simulink model "simpleVehicleModel_Trial1"  (R2017b)
settings: Solver=FixedStepAuto  StartTime=0.0  StopTime=15  FixedStep=0.01  RelTol=1e-3
values from neighbouring files (symbols this model uses):
  beta_ref = 20*pi/180    (= 0.349065850399)    [initialize_simplemodel_Trial.m]
  g = 9.81    [initialize_simplemodel.m]    (also in initialize_simplemodel_Trial.m; tire_friction_circle.m)
  h = 0.35    [initialize_simplemodel.m]    (also in initialize_simplemodel_Trial.m)
  Izz = 1800    [initialize_simplemodel.m]    (also in initialize_simplemodel_Trial.m = 1400)
  lf = 1.4    [initialize_simplemodel.m]    (also in initialize_simplemodel_Trial.m)
  lr = 1.345    [initialize_simplemodel.m]    (also in initialize_simplemodel_Trial.m)
  m = 1400    [initialize_simplemodel.m]    (also in initialize_simplemodel_Trial.m = 1300; tire_friction_circle.m = 1300)
  r = 0.34    [initialize_simplemodel.m]    (also in initialize_simplemodel_Trial.m)
  tr = 1.684/2    (= 0.842)    [initialize_simplemodel.m]    (also in initialize_simplemodel_Trial.m)
  vx = 10    [initialize_simplemodel_Trial.m]    (also in pp_from_simple_model.m; tire_friction_circle.m = 5)
undefined symbols (not defined in the file or in its folder): DiscIntNeverNeededParam, G1, G2
libraries: simulink x49
(part 1 of 2)
settings Model: Creator=ashwin.ramanujam  LastModifiedBy=gandh

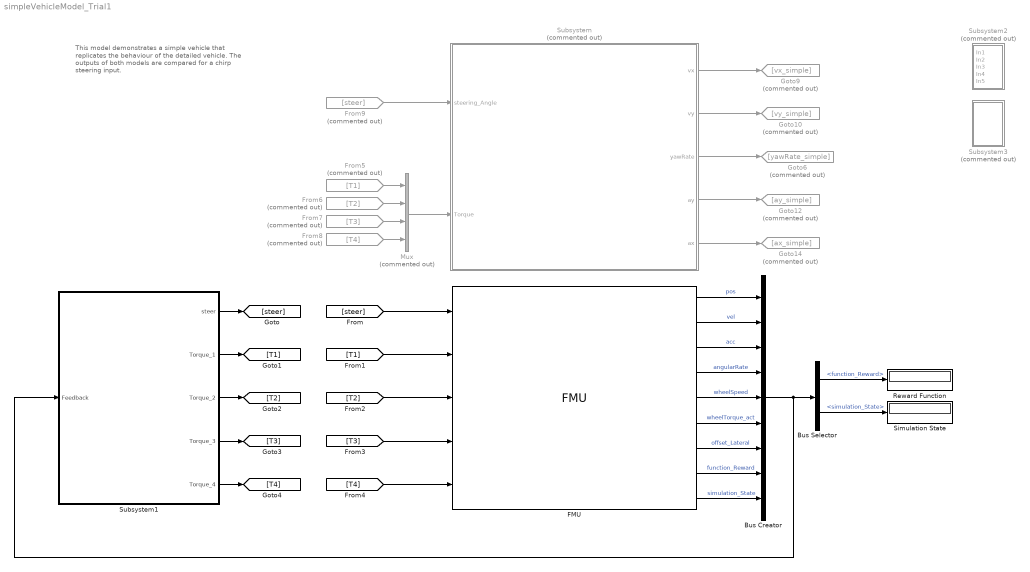
== system simpleVehicleModel_Trial1 ==
  note: This model demonstrates a simple vehicle that replicates the behaviour of the detailed vehicle. The outputs of both models are compared for a chirp steering input.
  Bus Creator : BusCreator  Inputs=9
  Bus Selector : BusSelector  OutputSignals=function_Reward,simulation_State
  FMU : FMU  FMUName=MED2018_VehicleModel.fmu  FMUMode=CoSimulation  FMUSampleTime=-1  mask(MED2018.VehicleModel [Co-Simulation, v2.0]){}
      mask Display:
      | if (exist([Simulink.fileGenControl('get','CacheFolder') '\slprj\_fmu\927a4232b314fe75ed86affe217e189d\MED2018_VehicleModel\model.png'],'file'))
      |     image([Simulink.fileGenControl('get','CacheFolder') '\slprj\_fmu\927a4232b314fe75ed86affe217e189d\MED2018_VehicleModel\model.png']);
      |     text(0.03, 0.97, 'MED2018.VehicleModel', 'horizontalAlignment', 'left', 'verticalAlignment', 'top');
      | else
      |     disp('MED2018.VehicleModel');
      | end
      | port_label('output',1,'Position');
      | port_label('output',2,'Velocity');
      | port_label('output',3,'Acceleration');
      | port_label('output',4,'angularRate');
      | port_label('output',5,'wheelSpeed');
      | port_label('output',6,'wheelTorque_act');
      | port_label('output',7,'offset_Lateral');
      | port_label('output',8,'function_Reward');
      | port_label('output',9,'simulation_State');
      | port_label('input',1,'steering_Angle');
      | port_label('input',2,'wheelTorque_cmd_FL');
      | port_label('input',3,'wheelTorque_cmd_FR');
      | port_label('input',4,'wheelTorque_cmd_RL');
      | port_label('input',5,'wheelTorque_cmd_RR');
  From5 : From  Commented=on  GotoTag=T1
  From6 : From  Commented=on  GotoTag=T2
  From7 : From  Commented=on  GotoTag=T3
  From8 : From  Commented=on  GotoTag=T4
  From9 : From  Commented=on  GotoTag=steer
  Goto10 : Goto  Commented=on  GotoTag=vy_simple
  Goto12 : Goto  Commented=on  GotoTag=ay_simple
  Goto14 : Goto  Commented=on  GotoTag=ax_simple
  Goto6 : Goto  Commented=on  GotoTag=yawRate_simple
  Goto9 : Goto  Commented=on  GotoTag=vx_simple
  Mux : Mux  Commented=on
  Reward Function : Display
  Simulation State : Display
  Subsystem : Subsystem  Commented=on
  Subsystem1 : Subsystem
  Subsystem2 : Subsystem  Commented=on
  Subsystem3 : Subsystem  Commented=on
  wires:
  Mux/1 -> Subsystem/2(Torque)
  [steer] -> FMU/1
  [T4] -> FMU/5
  [T1] -> FMU/2
  [T2] -> FMU/3
  [T3] -> FMU/4
  From5/1 -> Mux/1
  From6/1 -> Mux/2
  From7/1 -> Mux/3
  From8/1 -> Mux/4
  Subsystem/3(yawRate) -> Goto6/1
  Subsystem/1(vx) -> Goto9/1
  Subsystem/2(vy) -> Goto10/1
  Subsystem/4(ay) -> Goto12/1
  Subsystem/5(ax) -> Goto14/1
  From9/1 -> Subsystem/1(steering_Angle)
  Subsystem1/1(steer) -> [steer]
  Subsystem1/2(Torque_1) -> [T1]
  Subsystem1/3(Torque_2) -> [T2]
  Subsystem1/4(Torque_3) -> [T3]
  Subsystem1/5(Torque_4) -> [T4]
  FMU/1 -> Bus Creator/1  "pos"
  FMU/6 -> Bus Creator/6  "wheelTorque_act"
  FMU/8 -> Bus Creator/8  "function_Reward"
  FMU/3 -> Bus Creator/3  "acc"
  FMU/5 -> Bus Creator/5  "wheelSpeed"
  FMU/7 -> Bus Creator/7  "offset_Lateral"
  FMU/2 -> Bus Creator/2  "vel"
  FMU/4 -> Bus Creator/4  "angularRate"
  FMU/9 -> Bus Creator/9  "simulation_State"
  Bus Creator/1 -> Subsystem1/1(Feedback), Bus Selector/1
  Bus Selector/1 -> Reward Function/1  "<function_Reward>"
  Bus Selector/2 -> Simulation State/1  "<simulation_State>"

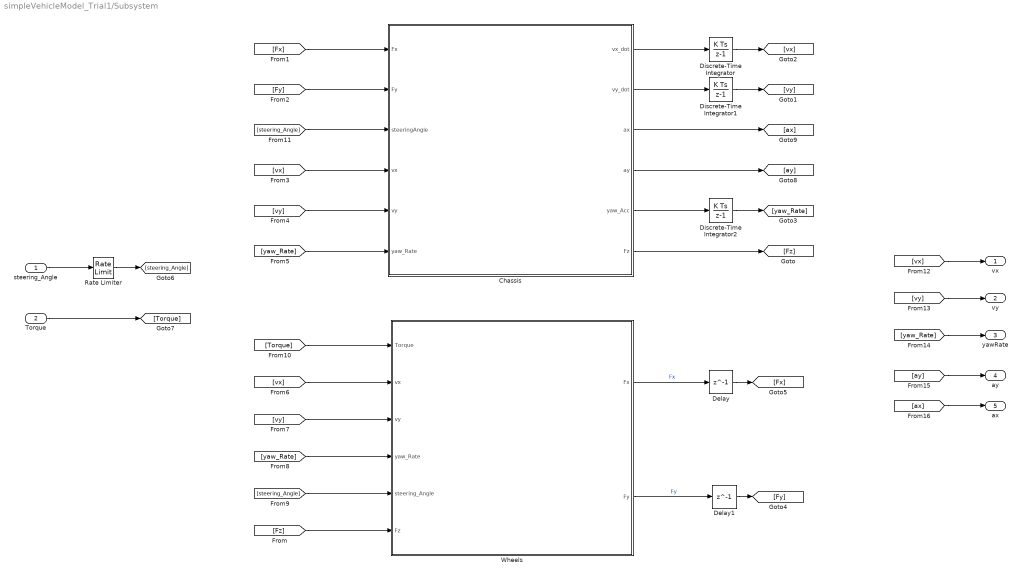
== system simpleVehicleModel_Trial1/Subsystem ==
  steering_Angle : Inport
  Torque : Inport  Port=2
  Chassis : MATLAB Function  TreatAsAtomicUnit=on
  Delay : Delay  DelayLength=1  InitialCondition=[m*g*lr/(lf+lr)/2;m*g*lr/(lf+lr)/2;m*g*lf/(lf+lr)/2;m*g*lf/(lf+lr)/2]
  Delay1 : Delay  DelayLength=1  InitialCondition=[m*g*lr/(lf+lr)/2;m*g*lr/(lf+lr)/2;m*g*lf/(lf+lr)/2;m*g*lf/(lf+lr)/2]
  Discrete-Time Integrator : DiscreteIntegrator  InitialCondition=60*5/18  InitialConditionSetting=State (most efficient)  SampleTime=-1  ICPrevOutput=DiscIntNeverNeededParam  ICPrevScaledInput=DiscIntNeverNeededParam
  Discrete-Time Integrator1 : DiscreteIntegrator  InitialConditionSetting=State (most efficient)  SampleTime=-1  ICPrevOutput=DiscIntNeverNeededParam  ICPrevScaledInput=DiscIntNeverNeededParam
  Discrete-Time Integrator2 : DiscreteIntegrator  InitialConditionSetting=State (most efficient)  SampleTime=-1  ICPrevOutput=DiscIntNeverNeededParam  ICPrevScaledInput=DiscIntNeverNeededParam
  Rate Limiter : RateLimiter  RisingSlewLimit=500*pi/180/12  FallingSlewLimit=-500*pi/180/12  SampleTimeMode=inherited
  Wheels : Subsystem  Priority=0
  vx : Outport
  vy : Outport  Port=2
  yawRate : Outport  Port=3
  ay : Outport  Port=4
  ax : Outport  Port=5
  wires:
  [vx] -> Chassis/4(vx)
  Discrete-Time Integrator2/1 -> [yaw_Rate]
  [Fy] -> Chassis/2(Fy)
  [vy] -> Wheels/3(vy)
  [Torque] -> Wheels/1(Torque)
  [yaw_Rate] -> yawRate/1
  [yaw_Rate] -> Wheels/4(yaw_Rate)
  [vx] -> vx/1
  [vx] -> Wheels/2(vx)
  [Fz] -> Wheels/6(Fz)
  [steering_Angle] -> Chassis/3(steeringAngle)
  [steering_Angle] -> Wheels/5(steering_Angle)
  steering_Angle/1 -> Rate Limiter/1
  Torque/1 -> [Torque]
  [vy] -> vy/1
  Chassis/5(yaw_Acc) -> Discrete-Time Integrator2/1
  Wheels/1(Fx) -> Delay/1  "Fx"
  Wheels/2(Fy) -> Delay1/1  "Fy"
  Chassis/6(Fz) -> [Fz]
  [ay] -> ay/1
  Delay/1 -> [Fx]
  Delay1/1 -> [Fy]
  Chassis/1(vx_dot) -> Discrete-Time Integrator/1
  Chassis/4(ay) -> [ay]
  Chassis/3(ax) -> [ax]
  [ax] -> ax/1
  Chassis/2(vy_dot) -> Discrete-Time Integrator1/1
  [vy] -> Chassis/5(vy)
  [yaw_Rate] -> Chassis/6(yaw_Rate)
  [Fx] -> Chassis/1(Fx)
  Discrete-Time Integrator1/1 -> [vy]
  Discrete-Time Integrator/1 -> [vx]
  Rate Limiter/1 -> [steering_Angle]

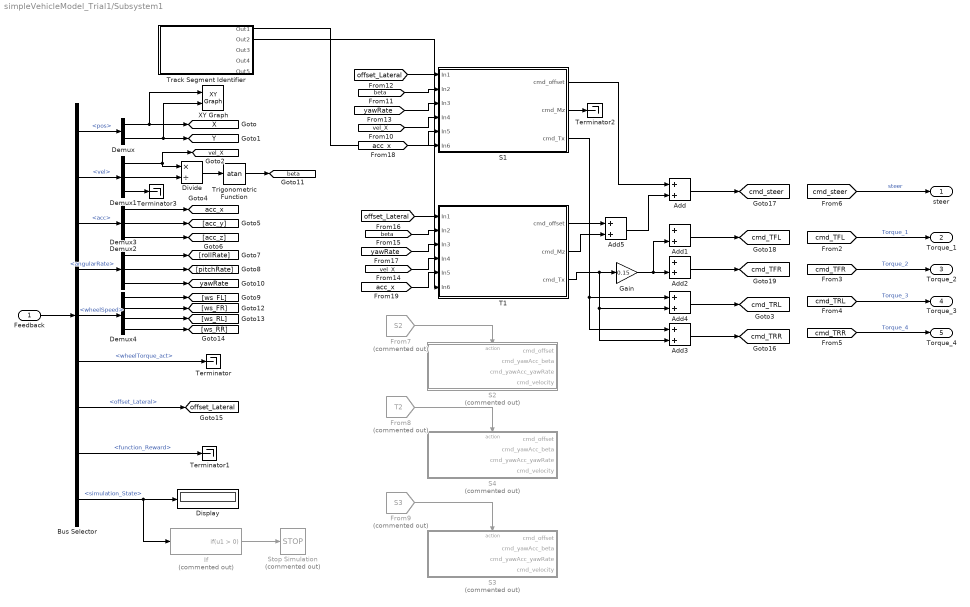
== system simpleVehicleModel_Trial1/Subsystem1 ==
  Feedback : Inport
  Add{,1..5} (6 alike) : Sum
  Bus Selector : BusSelector  OutputSignals=pos,vel,acc,angularRate,wheelSpeed,wheelTorque_act,offset_Lateral,function_Reward,simulation_State
  Demux : Demux  Outputs=2
  Demux1 : Demux  Outputs=3
  Demux2 : Demux  Outputs=3
  Demux3 : Demux  Outputs=3
  Demux4 : Demux
  Display : Display
  Divide : Product  Inputs=*/
  From7 : From  Commented=on  GotoTag=S2  TagVisibility=global
  From8 : From  Commented=on  GotoTag=T2  TagVisibility=global
  From9 : From  Commented=on  GotoTag=S3  TagVisibility=global
  Gain : Gain  Gain=0.15
  If : If  Commented=on  ShowElse=off
  S1 : Subsystem  TreatAsAtomicUnit=on
  S2 : Subsystem  Commented=on  TreatAsAtomicUnit=on
  S3 : Subsystem  Commented=on  TreatAsAtomicUnit=on
  S4 : Subsystem  Commented=on  TreatAsAtomicUnit=on
  Stop Simulation : Stop  Commented=on
  T1 : Subsystem  TreatAsAtomicUnit=on
  Terminator{,1..3} (4 alike) : Terminator
  Track Segment Identifier : Subsystem
  Trigonometric Function : Trigonometry  Operator=atan
  XY Graph : simulink/Sinks/XY Graph  xmin=-5  xmax=110  ymin=-10  ymax=180  st=-1
  steer : Outport
  Torque_1 : Outport  Port=2
  Torque_2 : Outport  Port=3
  Torque_3 : Outport  Port=4
  Torque_4 : Outport  Port=5
  tag scope: X=global, Y=global, acc_x=global, beta=global, cmd_TFL=global, cmd_TFR=global, cmd_TRL=global, cmd_TRR=global, cmd_steer=global, offset_Lateral=global, vel_X=global, yawRate=global
  wires:
  [cmd_TFL] -> Torque_1/1  "Torque_1"
  [cmd_TRL] -> Torque_3/1  "Torque_3"
  [cmd_TFR] -> Torque_2/1  "Torque_2"
  [cmd_TRR] -> Torque_4/1  "Torque_4"
  [cmd_steer] -> steer/1  "steer"
  Feedback/1 -> Bus Selector/1
  Bus Selector/1 -> Demux/1  "<pos>"
  Demux/2 -> XY Graph/2, [Y]
  Demux/1 -> XY Graph/1, [X]
  Demux1/1 -> Divide/1, [vel_X]
  Bus Selector/2 -> Demux1/1  "<vel>"
  Demux2/3 -> [acc_z]
  Bus Selector/3 -> Demux2/1  "<acc>"
  Demux2/2 -> [acc_y]
  Demux2/1 -> [acc_x]
  Demux3/1 -> [rollRate]
  Demux3/2 -> [pitchRate]
  Bus Selector/4 -> Demux3/1  "<angularRate>"
  Demux3/3 -> [yawRate]
  Demux4/3 -> [ws_RL]
  Bus Selector/5 -> Demux4/1  "<wheelSpeed>"
  Demux4/2 -> [ws_FR]
  Demux4/1 -> [ws_FL]
  Demux4/4 -> [ws_RR]
  Bus Selector/6 -> Terminator/1  "<wheelTorque_act>"
  Bus Selector/7 -> [offset_Lateral]  "<offset_Lateral>"
  Bus Selector/8 -> Terminator1/1  "<function_Reward>"
  Bus Selector/9 -> If/1, Display/1  "<simulation_State>"
  Demux1/2 -> Divide/2
  Divide/1 -> Trigonometric Function/1
  Trigonometric Function/1 -> [beta]
  If/1 -> Stop Simulation/1
  From7/1 -> S2/Action
  From8/1 -> S4/Action
  From9/1 -> S3/Action
  Add/1 -> [cmd_steer]
  Add1/1 -> [cmd_TFL]
  Add2/1 -> [cmd_TFR]
  Add4/1 -> [cmd_TRL]
  Add3/1 -> [cmd_TRR]
  S1/1(cmd_offset) -> Add/1
  T1/3(cmd_Tx) -> Gain/1, Add4/2, Add3/2
  Add5/1 -> Add/2
  T1/2(cmd_Mz) -> Add5/2
  T1/1(cmd_offset) -> Add5/1
  S1/3(cmd_Tx) -> Add3/1, Add4/1
  S1/2(cmd_Mz) -> Terminator2/1
  Gain/1 -> Add1/2, Add2/2
  Demux1/3 -> Terminator3/1
  [vel_X] -> S1/4(In4)
  [beta] -> S1/2(In2)
  [offset_Lateral] -> S1/1(In1)
  [yawRate] -> S1/3(In3)
  [yawRate] -> T1/3(In3)
  [offset_Lateral] -> T1/1(In1)
  [beta] -> T1/2(In2)
  [vel_X] -> T1/4(In4)
  [acc_x] -> S1/5(In5)
  [acc_x] -> T1/5(In5)
  Track Segment Identifier/1(Out1) -> S1/6(In6)
  Track Segment Identifier/2(Out2) -> T1/6(In6)

== system simpleVehicleModel_Trial1/Subsystem2 ==
  In1 : Inport
  In2 : Inport  Port=2
  In3 : Inport  Port=3
  In4 : Inport  Port=4
  In5 : Inport  Port=5
  Demux : Demux  Commented=on  Outputs=3
  Demux1 : Demux  Commented=on  Outputs=3
  Demux2 : Demux  Commented=on  Outputs=3
  Demux3 : Demux  Commented=on  Outputs=2
  Goto11 : Goto  Commented=on  GotoTag=ay_FMU
  Goto13 : Goto  Commented=on  GotoTag=ax_FMU
  Goto15 : Goto  Commented=on  GotoTag=offset_Lateral  TagVisibility=global
  Goto5 : Goto  Commented=on  GotoTag=yawRate_FMU
  Goto7 : Goto  Commented=on  GotoTag=vx_FMU
  Goto8 : Goto  Commented=on  GotoTag=vy_FMU
  Terminator{,2..4} (4 alike) : Terminator  Commented=on
  XY Graph : simulink/Sinks/XY Graph  Commented=on  xmin=-5  xmax=110  ymin=-10  ymax=180  st=-1
  wires:
  Demux/3 -> Goto5/1
  Demux1/1 -> Goto7/1
  Demux1/2 -> Goto8/1
  Demux/1 -> Terminator3/1
  Demux/2 -> Terminator4/1
  Demux2/2 -> Goto11/1
  Demux1/3 -> Terminator/1
  Demux2/1 -> Goto13/1
  Demux3/1 -> XY Graph/1
  Demux3/2 -> XY Graph/2
  Demux2/3 -> Terminator2/1
  In5/1 -> Goto15/1
  In2/1 -> Demux1/1
  In4/1 -> Demux/1
  In1/1 -> Demux3/1
  In3/1 -> Demux2/1

== system simpleVehicleModel_Trial1/Subsystem3 ==
  Scope{,1..3,5} (5 alike) : Scope  NumInputPorts=2
  wires:
  [vx_simple] -> Scope/1  "vx_simple"
  [vx_FMU] -> Scope/2  "vx_FMU"
  [vy_FMU] -> Scope1/2  "vy_FMU"
  [vy_simple] -> Scope1/1  "vy_simple"
  [ax_FMU] -> Scope5/2  "ax_FMU"
  [yawRate_simple] -> Scope2/1  "yawRate_simple"
  [yawRate_FMU] -> Scope2/2  "yawRate_FMU"
  [ay_simple] -> Scope3/1  "ay_simple"
  [ay_FMU] -> Scope3/2  "ay_FMU"
  [ax_simple] -> Scope5/1  "ax_simple"

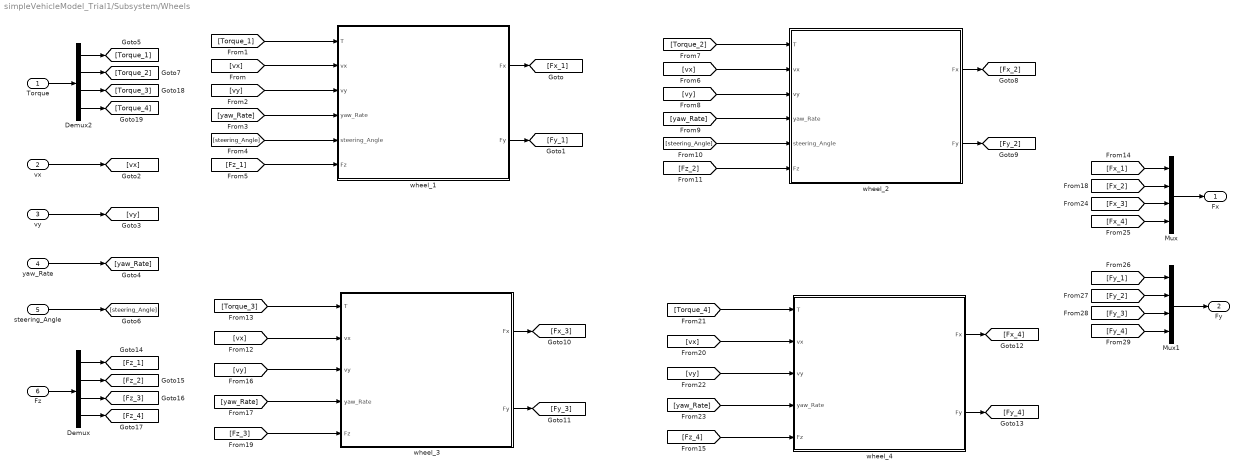
== system simpleVehicleModel_Trial1/Subsystem/Wheels ==
  Torque : Inport
  vx : Inport  Port=2
  vy : Inport  Port=3
  yaw_Rate : Inport  Port=4
  steering_Angle : Inport  Port=5
  Fz : Inport  Port=6
  Demux : Demux
  Demux2 : Demux
  Mux : Mux
  Mux1 : Mux
  wheel_1 : Subsystem
  wheel_2 : Subsystem
  wheel_3 : Subsystem
  wheel_4 : Subsystem
  Fx : Outport
  Fy : Outport  Port=2
  wires:
  vx/1 -> [vx]
  vy/1 -> [vy]
  yaw_Rate/1 -> [yaw_Rate]
  [vx] -> wheel_1/2(vx)
  wheel_1/1(Fx) -> [Fx_1]
  wheel_1/2(Fy) -> [Fy_1]
  [steering_Angle] -> wheel_1/5(steering_Angle)
  [yaw_Rate] -> wheel_1/4(yaw_Rate)
  [vy] -> wheel_1/3(vy)
  [Torque_1] -> wheel_1/1(T)
  steering_Angle/1 -> [steering_Angle]
  wheel_2/1(Fx) -> [Fx_2]
  wheel_2/2(Fy) -> [Fy_2]
  [yaw_Rate] -> wheel_2/4(yaw_Rate)
  [vy] -> wheel_2/3(vy)
  [steering_Angle] -> wheel_2/5(steering_Angle)
  [vx] -> wheel_2/2(vx)
  wheel_3/1(Fx) -> [Fx_3]
  [yaw_Rate] -> wheel_3/4(yaw_Rate)
  [vy] -> wheel_4/3(vy)
  [yaw_Rate] -> wheel_4/4(yaw_Rate)
  [vx] -> wheel_4/2(vx)
  wheel_4/2(Fy) -> [Fy_4]
  wheel_3/2(Fy) -> [Fy_3]
  wheel_4/1(Fx) -> [Fx_4]
  [vy] -> wheel_3/3(vy)
  [vx] -> wheel_3/2(vx)
  [Fx_1] -> Mux/1
  [Fx_2] -> Mux/2
  [Fx_3] -> Mux/3
  [Fx_4] -> Mux/4
  [Fy_3] -> Mux1/3
  [Fy_4] -> Mux1/4
  [Fy_2] -> Mux1/2
  [Fy_1] -> Mux1/1
  Demux/1 -> [Fz_1]
  Demux/2 -> [Fz_2]
  Demux/3 -> [Fz_3]
  Demux/4 -> [Fz_4]
  [Fz_1] -> wheel_1/6(Fz)
  [Fz_3] -> wheel_3/5(Fz)
  [Fz_4] -> wheel_4/5(Fz)
  [Fz_2] -> wheel_2/6(Fz)
  Fz/1 -> Demux/1
  [Torque_3] -> wheel_3/1(T)
  [Torque_2] -> wheel_2/1(T)
  [Torque_4] -> wheel_4/1(T)
  Demux2/4 -> [Torque_4]
  Demux2/3 -> [Torque_3]
  Demux2/1 -> [Torque_1]
  Torque/1 -> Demux2/1
  Demux2/2 -> [Torque_2]
  Mux1/1 -> Fy/1
  Mux/1 -> Fx/1

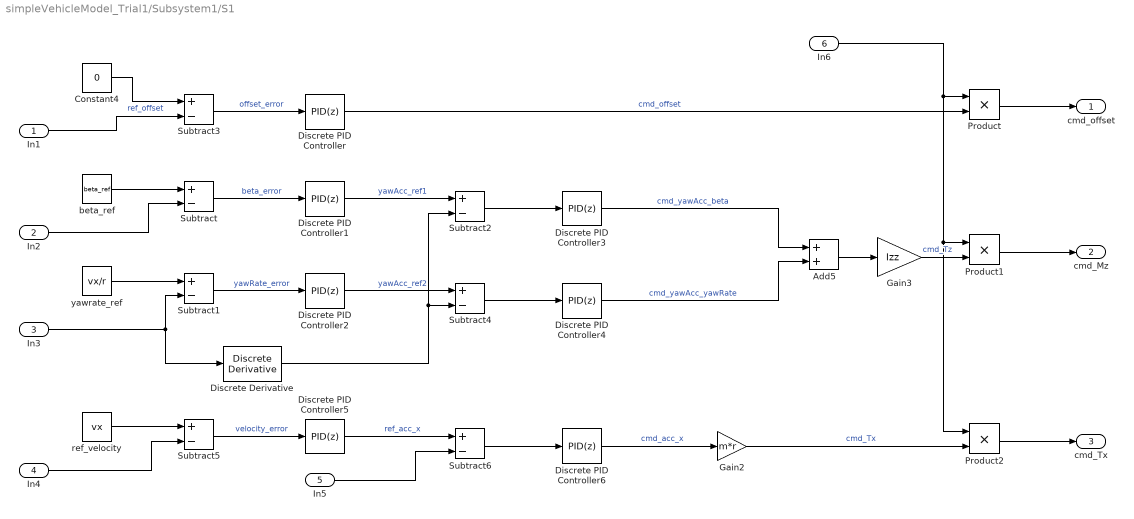
== system simpleVehicleModel_Trial1/Subsystem1/S1 ==
  In1 : Inport
  In2 : Inport  Port=2
  In3 : Inport  Port=3
  In4 : Inport  Port=4
  In5 : Inport  Port=5
  In6 : Inport  Port=6
  Add5 : Sum
  Constant4 : Constant  Value=0
  Discrete Derivative : simulink/Discrete/Discrete Derivative  gainval=1.0  ICPrevScaledInput=0.0  OutMin=[]  OutMax=[]  OutDataType=fixdt(1, 16)  OutScaling=2^-10  DoSatur=off
  Discrete PID Controller : simulink/Continuous/PID Controller  Controller=PID  TimeDomain=Discrete-time  SampleTime=-1  IntegratorMethod=Forward Euler  FilterMethod=Forward Euler  Form=Parallel  UseFilter=on  ControllerParametersSource=internal  P=1  I=0  D=0.1  N=100  InitialConditionSource=internal  InitialConditionForIntegrator=0  InitialConditionForFilter=0  ExternalReset=none  LimitOutput=off  UpperSaturationLimit=inf  LowerSaturationLimit=-inf  LinearizeAsGain=off  AntiWindupMode=none  Kb=1  TrackingMode=off  Kt=1  PParamMin=[]  PParamMax=[]  IParamMin=[]  IParamMax=[]  DParamMin=[]  DParamMax=[]  NParamMin=[]  NParamMax=[]  KbParamMin=[]  KbParamMax=[]  KtParamMin=[]  KtParamMax=[]  POutMin=[]  POutMax=[]  IOutMin=[]  IOutMax=[]  DOutMin=[]  DOutMax=[]  NOutMin=[]  NOutMax=[]  KbOutMin=[]  KbOutMax=[]  KtOutMin=[]  KtOutMax=[]  IntegratorOutMin=[]  IntegratorOutMax=[]  FilterOutMin=[]  FilterOutMax=[]  SumOutMin=[]  SumOutMax=[]  SumI1OutMin=[]  SumI1OutMax=[]  SumI2OutMin=[]  SumI2OutMax=[]  SumI3OutMin=[]  SumI3OutMax=[]  SumDOutMin=[]  SumDOutMax=[]  SaturationOutMin=[]  SaturationOutMax=[]  IntegratorContinuousStateAttributes=''  IntegratorStateMustResolveToSignalObject=off  IntegratorRTWStateStorageClass=Auto  FilterContinuousStateAttributes=''  FilterStateMustResolveToSignalObject=off  FilterRTWStateStorageClass=Auto  DifferentiatorICPrevScaledInput=0  DifferentiatorOutMin=[]  DifferentiatorOutMax=[]  InitialConditionSetting=State (most efficient)  FilterDiffOutCoefMin=[]  FilterDiffOutCoefMax=[]  SumDenOutMin=[]  SumDenOutMax=[]  SumNumOutMin=[]  SumNumOutMax=[]  ReciprocalOutMin=[]  ReciprocalOutMax=[]  DivideOutMin=[]  DivideOutMax=[]  TunerSelectOption=Transfer Function Based (PID Tuner App)
  Discrete PID Controller{1..6} (6 alike) : simulink/Continuous/PID Controller  Controller=PID  TimeDomain=Discrete-time  SampleTime=-1  IntegratorMethod=Forward Euler  FilterMethod=Forward Euler  Form=Parallel  UseFilter=on  ControllerParametersSource=internal  P=1  I=1  D=0  N=100  InitialConditionSource=internal  InitialConditionForIntegrator=0  InitialConditionForFilter=0  ExternalReset=none  LimitOutput=off  UpperSaturationLimit=inf  LowerSaturationLimit=-inf  LinearizeAsGain=off  AntiWindupMode=none  Kb=1  TrackingMode=off  Kt=1  PParamMin=[]  PParamMax=[]  IParamMin=[]  IParamMax=[]  DParamMin=[]  DParamMax=[]  NParamMin=[]  NParamMax=[]  KbParamMin=[]  KbParamMax=[]  KtParamMin=[]  KtParamMax=[]  POutMin=[]  POutMax=[]  IOutMin=[]  IOutMax=[]  DOutMin=[]  DOutMax=[]  NOutMin=[]  NOutMax=[]  KbOutMin=[]  KbOutMax=[]  KtOutMin=[]  KtOutMax=[]  IntegratorOutMin=[]  IntegratorOutMax=[]  FilterOutMin=[]  FilterOutMax=[]  SumOutMin=[]  SumOutMax=[]  SumI1OutMin=[]  SumI1OutMax=[]  SumI2OutMin=[]  SumI2OutMax=[]  SumI3OutMin=[]  SumI3OutMax=[]  SumDOutMin=[]  SumDOutMax=[]  SaturationOutMin=[]  SaturationOutMax=[]  IntegratorContinuousStateAttributes=''  IntegratorStateMustResolveToSignalObject=off  IntegratorRTWStateStorageClass=Auto  FilterContinuousStateAttributes=''  FilterStateMustResolveToSignalObject=off  FilterRTWStateStorageClass=Auto  DifferentiatorICPrevScaledInput=0  DifferentiatorOutMin=[]  DifferentiatorOutMax=[]  InitialConditionSetting=State (most efficient)  FilterDiffOutCoefMin=[]  FilterDiffOutCoefMax=[]  SumDenOutMin=[]  SumDenOutMax=[]  SumNumOutMin=[]  SumNumOutMax=[]  ReciprocalOutMin=[]  ReciprocalOutMax=[]  DivideOutMin=[]  DivideOutMax=[]  TunerSelectOption=Transfer Function Based (PID Tuner App)
  Gain2 : Gain  Gain=m*r
  Gain3 : Gain  Gain=Izz
  Product : Product
  Product1 : Product
  Product2 : Product
  Subtract{,1..6} (7 alike) : Sum  Inputs=+-
  beta_ref : Constant  Value=beta_ref
  ref_velocity : Constant  Value=vx
  yawrate_ref : Constant  Value=vx/r
  cmd_offset : Outport
  cmd_Mz : Outport  Port=2
  cmd_Tx : Outport  Port=3
  wires:
  Discrete PID Controller6/1 -> Gain2/1  "cmd_acc_x"
  In5/1 -> Subtract6/2
  Subtract6/1 -> Discrete PID Controller6/1
  Add5/1 -> Gain3/1
  Discrete PID Controller5/1 -> Subtract6/1  "ref_acc_x"
  Subtract5/1 -> Discrete PID Controller5/1  "velocity_error"
  ref_velocity/1 -> Subtract5/1
  In4/1 -> Subtract5/2
  Discrete Derivative/1 -> Subtract2/2, Subtract4/2
  Constant4/1 -> Subtract3/1  "ref_offset"
  Discrete PID Controller3/1 -> Add5/1  "cmd_yawAcc_beta"
  Subtract/1 -> Discrete PID Controller1/1  "beta_error"
  Subtract4/1 -> Discrete PID Controller4/1
  beta_ref/1 -> Subtract/1
  Discrete PID Controller2/1 -> Subtract4/1  "yawAcc_ref2"
  Subtract3/1 -> Discrete PID Controller/1  "offset_error"
  In3/1 -> Subtract1/2, Discrete Derivative/1
  Discrete PID Controller1/1 -> Subtract2/1  "yawAcc_ref1"
  yawrate_ref/1 -> Subtract1/1
  Subtract2/1 -> Discrete PID Controller3/1
  In1/1 -> Subtract3/2
  In2/1 -> Subtract/2
  Subtract1/1 -> Discrete PID Controller2/1  "yawRate_error"
  Discrete PID Controller4/1 -> Add5/2  "cmd_yawAcc_yawRate"
  Product/1 -> cmd_offset/1
  Discrete PID Controller/1 -> Product/2  "cmd_offset"
  Product1/1 -> cmd_Mz/1
  Gain3/1 -> Product1/2  "cmd_Tz"
  Product2/1 -> cmd_Tx/1
  Gain2/1 -> Product2/2  "cmd_Tx"
  In6/1 -> Product/1, Product2/1, Product1/1

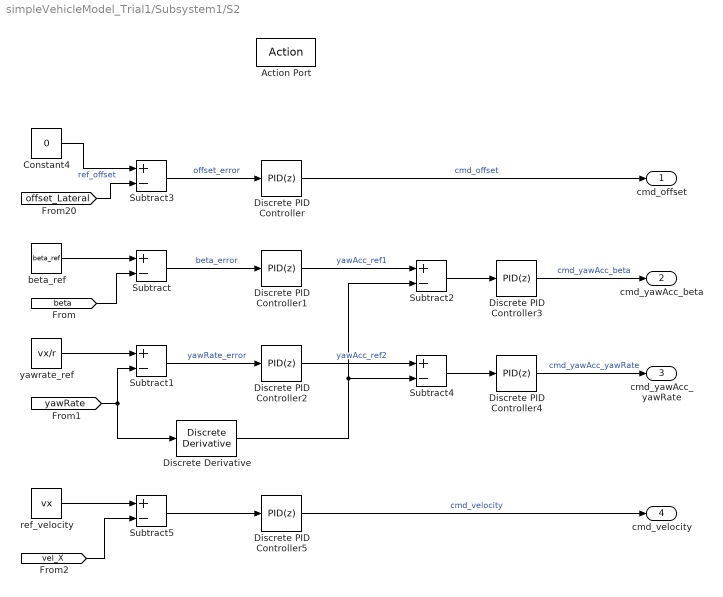
== system simpleVehicleModel_Trial1/Subsystem1/S2 ==
  Action Port : ActionPort
  Constant4 : Constant  Value=0
  Discrete Derivative : simulink/Discrete/Discrete Derivative  gainval=1.0  ICPrevScaledInput=0.0  OutMin=[]  OutMax=[]  OutDataType=fixdt(1, 16)  OutScaling=2^-10  DoSatur=off
  Discrete PID Controller : simulink/Continuous/PID Controller  Controller=PID  TimeDomain=Discrete-time  SampleTime=-1  IntegratorMethod=Forward Euler  FilterMethod=Forward Euler  Form=Parallel  UseFilter=on  ControllerParametersSource=internal  P=1  I=0  D=0.1  N=100  InitialConditionSource=internal  InitialConditionForIntegrator=0  InitialConditionForFilter=0  ExternalReset=none  LimitOutput=off  UpperSaturationLimit=inf  LowerSaturationLimit=-inf  LinearizeAsGain=off  AntiWindupMode=none  Kb=1  TrackingMode=off  Kt=1  PParamMin=[]  PParamMax=[]  IParamMin=[]  IParamMax=[]  DParamMin=[]  DParamMax=[]  NParamMin=[]  NParamMax=[]  KbParamMin=[]  KbParamMax=[]  KtParamMin=[]  KtParamMax=[]  POutMin=[]  POutMax=[]  IOutMin=[]  IOutMax=[]  DOutMin=[]  DOutMax=[]  NOutMin=[]  NOutMax=[]  KbOutMin=[]  KbOutMax=[]  KtOutMin=[]  KtOutMax=[]  IntegratorOutMin=[]  IntegratorOutMax=[]  FilterOutMin=[]  FilterOutMax=[]  SumOutMin=[]  SumOutMax=[]  SumI1OutMin=[]  SumI1OutMax=[]  SumI2OutMin=[]  SumI2OutMax=[]  SumI3OutMin=[]  SumI3OutMax=[]  SumDOutMin=[]  SumDOutMax=[]  SaturationOutMin=[]  SaturationOutMax=[]  IntegratorContinuousStateAttributes=''  IntegratorStateMustResolveToSignalObject=off  IntegratorRTWStateStorageClass=Auto  FilterContinuousStateAttributes=''  FilterStateMustResolveToSignalObject=off  FilterRTWStateStorageClass=Auto  DifferentiatorICPrevScaledInput=0  DifferentiatorOutMin=[]  DifferentiatorOutMax=[]  InitialConditionSetting=State (most efficient)  FilterDiffOutCoefMin=[]  FilterDiffOutCoefMax=[]  SumDenOutMin=[]  SumDenOutMax=[]  SumNumOutMin=[]  SumNumOutMax=[]  ReciprocalOutMin=[]  ReciprocalOutMax=[]  DivideOutMin=[]  DivideOutMax=[]  TunerSelectOption=Transfer Function Based (PID Tuner App)
  Discrete PID Controller{1..5} (5 alike) : simulink/Continuous/PID Controller  Controller=PID  TimeDomain=Discrete-time  SampleTime=-1  IntegratorMethod=Forward Euler  FilterMethod=Forward Euler  Form=Parallel  UseFilter=on  ControllerParametersSource=internal  P=1  I=1  D=0  N=100  InitialConditionSource=internal  InitialConditionForIntegrator=0  InitialConditionForFilter=0  ExternalReset=none  LimitOutput=off  UpperSaturationLimit=inf  LowerSaturationLimit=-inf  LinearizeAsGain=off  AntiWindupMode=none  Kb=1  TrackingMode=off  Kt=1  PParamMin=[]  PParamMax=[]  IParamMin=[]  IParamMax=[]  DParamMin=[]  DParamMax=[]  NParamMin=[]  NParamMax=[]  KbParamMin=[]  KbParamMax=[]  KtParamMin=[]  KtParamMax=[]  POutMin=[]  POutMax=[]  IOutMin=[]  IOutMax=[]  DOutMin=[]  DOutMax=[]  NOutMin=[]  NOutMax=[]  KbOutMin=[]  KbOutMax=[]  KtOutMin=[]  KtOutMax=[]  IntegratorOutMin=[]  IntegratorOutMax=[]  FilterOutMin=[]  FilterOutMax=[]  SumOutMin=[]  SumOutMax=[]  SumI1OutMin=[]  SumI1OutMax=[]  SumI2OutMin=[]  SumI2OutMax=[]  SumI3OutMin=[]  SumI3OutMax=[]  SumDOutMin=[]  SumDOutMax=[]  SaturationOutMin=[]  SaturationOutMax=[]  IntegratorContinuousStateAttributes=''  IntegratorStateMustResolveToSignalObject=off  IntegratorRTWStateStorageClass=Auto  FilterContinuousStateAttributes=''  FilterStateMustResolveToSignalObject=off  FilterRTWStateStorageClass=Auto  DifferentiatorICPrevScaledInput=0  DifferentiatorOutMin=[]  DifferentiatorOutMax=[]  InitialConditionSetting=State (most efficient)  FilterDiffOutCoefMin=[]  FilterDiffOutCoefMax=[]  SumDenOutMin=[]  SumDenOutMax=[]  SumNumOutMin=[]  SumNumOutMax=[]  ReciprocalOutMin=[]  ReciprocalOutMax=[]  DivideOutMin=[]  DivideOutMax=[]  TunerSelectOption=Transfer Function Based (PID Tuner App)
  Subtract{,1..5} (6 alike) : Sum  Inputs=+-
  beta_ref : Constant  Value=beta_ref
  ref_velocity : Constant  Value=vx
  yawrate_ref : Constant  Value=vx/r
  cmd_offset : Outport
  cmd_yawAcc_beta : Outport  Port=2
  cmd_yawAcc_yawRate : Outport  Port=3
  cmd_velocity : Outport  Port=4
  wires:
  Discrete PID Controller5/1 -> cmd_velocity/1  "cmd_velocity"
  Subtract5/1 -> Discrete PID Controller5/1
  ref_velocity/1 -> Subtract5/1
  [vel_X] -> Subtract5/2
  Discrete Derivative/1 -> Subtract2/2, Subtract4/2
  Constant4/1 -> Subtract3/1  "ref_offset"
  Discrete PID Controller3/1 -> cmd_yawAcc_beta/1  "cmd_yawAcc_beta"
  Subtract/1 -> Discrete PID Controller1/1  "beta_error"
  Subtract4/1 -> Discrete PID Controller4/1
  beta_ref/1 -> Subtract/1
  Discrete PID Controller2/1 -> Subtract4/1  "yawAcc_ref2"
  Subtract3/1 -> Discrete PID Controller/1  "offset_error"
  [yawRate] -> Subtract1/2, Discrete Derivative/1
  Discrete PID Controller1/1 -> Subtract2/1  "yawAcc_ref1"
  yawrate_ref/1 -> Subtract1/1
  Subtract2/1 -> Discrete PID Controller3/1
  [offset_Lateral] -> Subtract3/2
  Discrete PID Controller/1 -> cmd_offset/1  "cmd_offset"
  [beta] -> Subtract/2
  Subtract1/1 -> Discrete PID Controller2/1  "yawRate_error"
  Discrete PID Controller4/1 -> cmd_yawAcc_yawRate/1  "cmd_yawAcc_yawRate"

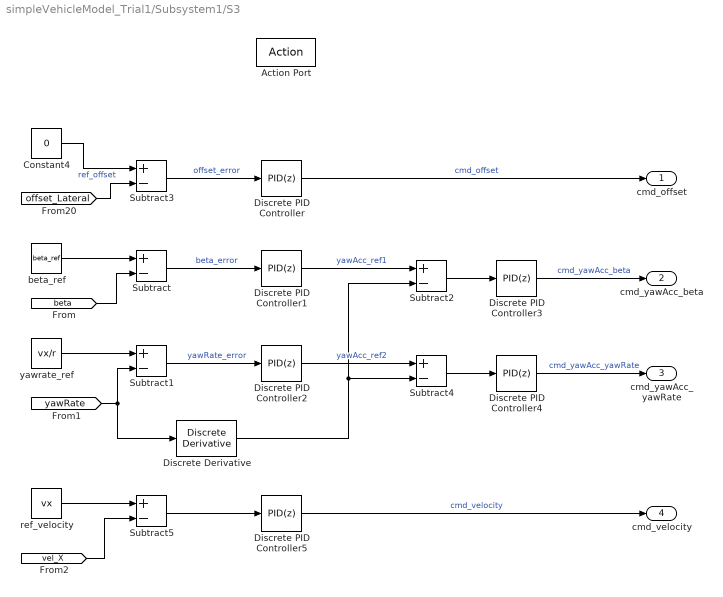
== system simpleVehicleModel_Trial1/Subsystem1/S3 ==
  Action Port : ActionPort
  Constant4 : Constant  Value=0
  Discrete Derivative : simulink/Discrete/Discrete Derivative  gainval=1.0  ICPrevScaledInput=0.0  OutMin=[]  OutMax=[]  OutDataType=fixdt(1, 16)  OutScaling=2^-10  DoSatur=off
  Discrete PID Controller : simulink/Continuous/PID Controller  Controller=PID  TimeDomain=Discrete-time  SampleTime=-1  IntegratorMethod=Forward Euler  FilterMethod=Forward Euler  Form=Parallel  UseFilter=on  ControllerParametersSource=internal  P=1  I=0  D=0.1  N=100  InitialConditionSource=internal  InitialConditionForIntegrator=0  InitialConditionForFilter=0  ExternalReset=none  LimitOutput=off  UpperSaturationLimit=inf  LowerSaturationLimit=-inf  LinearizeAsGain=off  AntiWindupMode=none  Kb=1  TrackingMode=off  Kt=1  PParamMin=[]  PParamMax=[]  IParamMin=[]  IParamMax=[]  DParamMin=[]  DParamMax=[]  NParamMin=[]  NParamMax=[]  KbParamMin=[]  KbParamMax=[]  KtParamMin=[]  KtParamMax=[]  POutMin=[]  POutMax=[]  IOutMin=[]  IOutMax=[]  DOutMin=[]  DOutMax=[]  NOutMin=[]  NOutMax=[]  KbOutMin=[]  KbOutMax=[]  KtOutMin=[]  KtOutMax=[]  IntegratorOutMin=[]  IntegratorOutMax=[]  FilterOutMin=[]  FilterOutMax=[]  SumOutMin=[]  SumOutMax=[]  SumI1OutMin=[]  SumI1OutMax=[]  SumI2OutMin=[]  SumI2OutMax=[]  SumI3OutMin=[]  SumI3OutMax=[]  SumDOutMin=[]  SumDOutMax=[]  SaturationOutMin=[]  SaturationOutMax=[]  IntegratorContinuousStateAttributes=''  IntegratorStateMustResolveToSignalObject=off  IntegratorRTWStateStorageClass=Auto  FilterContinuousStateAttributes=''  FilterStateMustResolveToSignalObject=off  FilterRTWStateStorageClass=Auto  DifferentiatorICPrevScaledInput=0  DifferentiatorOutMin=[]  DifferentiatorOutMax=[]  InitialConditionSetting=State (most efficient)  FilterDiffOutCoefMin=[]  FilterDiffOutCoefMax=[]  SumDenOutMin=[]  SumDenOutMax=[]  SumNumOutMin=[]  SumNumOutMax=[]  ReciprocalOutMin=[]  ReciprocalOutMax=[]  DivideOutMin=[]  DivideOutMax=[]  TunerSelectOption=Transfer Function Based (PID Tuner App)
  Discrete PID Controller{1..5} (5 alike) : simulink/Continuous/PID Controller  Controller=PID  TimeDomain=Discrete-time  SampleTime=-1  IntegratorMethod=Forward Euler  FilterMethod=Forward Euler  Form=Parallel  UseFilter=on  ControllerParametersSource=internal  P=1  I=1  D=0  N=100  InitialConditionSource=internal  InitialConditionForIntegrator=0  InitialConditionForFilter=0  ExternalReset=none  LimitOutput=off  UpperSaturationLimit=inf  LowerSaturationLimit=-inf  LinearizeAsGain=off  AntiWindupMode=none  Kb=1  TrackingMode=off  Kt=1  PParamMin=[]  PParamMax=[]  IParamMin=[]  IParamMax=[]  DParamMin=[]  DParamMax=[]  NParamMin=[]  NParamMax=[]  KbParamMin=[]  KbParamMax=[]  KtParamMin=[]  KtParamMax=[]  POutMin=[]  POutMax=[]  IOutMin=[]  IOutMax=[]  DOutMin=[]  DOutMax=[]  NOutMin=[]  NOutMax=[]  KbOutMin=[]  KbOutMax=[]  KtOutMin=[]  KtOutMax=[]  IntegratorOutMin=[]  IntegratorOutMax=[]  FilterOutMin=[]  FilterOutMax=[]  SumOutMin=[]  SumOutMax=[]  SumI1OutMin=[]  SumI1OutMax=[]  SumI2OutMin=[]  SumI2OutMax=[]  SumI3OutMin=[]  SumI3OutMax=[]  SumDOutMin=[]  SumDOutMax=[]  SaturationOutMin=[]  SaturationOutMax=[]  IntegratorContinuousStateAttributes=''  IntegratorStateMustResolveToSignalObject=off  IntegratorRTWStateStorageClass=Auto  FilterContinuousStateAttributes=''  FilterStateMustResolveToSignalObject=off  FilterRTWStateStorageClass=Auto  DifferentiatorICPrevScaledInput=0  DifferentiatorOutMin=[]  DifferentiatorOutMax=[]  InitialConditionSetting=State (most efficient)  FilterDiffOutCoefMin=[]  FilterDiffOutCoefMax=[]  SumDenOutMin=[]  SumDenOutMax=[]  SumNumOutMin=[]  SumNumOutMax=[]  ReciprocalOutMin=[]  ReciprocalOutMax=[]  DivideOutMin=[]  DivideOutMax=[]  TunerSelectOption=Transfer Function Based (PID Tuner App)
  Subtract{,1..5} (6 alike) : Sum  Inputs=+-
  beta_ref : Constant  Value=beta_ref
  ref_velocity : Constant  Value=vx
  yawrate_ref : Constant  Value=vx/r
  cmd_offset : Outport
  cmd_yawAcc_beta : Outport  Port=2
  cmd_yawAcc_yawRate : Outport  Port=3
  cmd_velocity : Outport  Port=4
  wires:
  Discrete PID Controller5/1 -> cmd_velocity/1  "cmd_velocity"
  Subtract5/1 -> Discrete PID Controller5/1
  ref_velocity/1 -> Subtract5/1
  [vel_X] -> Subtract5/2
  Discrete Derivative/1 -> Subtract2/2, Subtract4/2
  Constant4/1 -> Subtract3/1  "ref_offset"
  Discrete PID Controller3/1 -> cmd_yawAcc_beta/1  "cmd_yawAcc_beta"
  Subtract/1 -> Discrete PID Controller1/1  "beta_error"
  Subtract4/1 -> Discrete PID Controller4/1
  beta_ref/1 -> Subtract/1
  Discrete PID Controller2/1 -> Subtract4/1  "yawAcc_ref2"
  Subtract3/1 -> Discrete PID Controller/1  "offset_error"
  [yawRate] -> Subtract1/2, Discrete Derivative/1
  Discrete PID Controller1/1 -> Subtract2/1  "yawAcc_ref1"
  yawrate_ref/1 -> Subtract1/1
  Subtract2/1 -> Discrete PID Controller3/1
  [offset_Lateral] -> Subtract3/2
  Discrete PID Controller/1 -> cmd_offset/1  "cmd_offset"
  [beta] -> Subtract/2
  Subtract1/1 -> Discrete PID Controller2/1  "yawRate_error"
  Discrete PID Controller4/1 -> cmd_yawAcc_yawRate/1  "cmd_yawAcc_yawRate"

== system simpleVehicleModel_Trial1/Subsystem1/S4 ==
  Action Port : ActionPort
  Constant4 : Constant  Value=0
  Discrete Derivative : simulink/Discrete/Discrete Derivative  gainval=1.0  ICPrevScaledInput=0.0  OutMin=[]  OutMax=[]  OutDataType=fixdt(1, 16)  OutScaling=2^-10  DoSatur=off
  Discrete PID Controller : simulink/Continuous/PID Controller  Controller=PID  TimeDomain=Discrete-time  SampleTime=-1  IntegratorMethod=Forward Euler  FilterMethod=Forward Euler  Form=Parallel  UseFilter=on  ControllerParametersSource=internal  P=1  I=0  D=0.1  N=100  InitialConditionSource=internal  InitialConditionForIntegrator=0  InitialConditionForFilter=0  ExternalReset=none  LimitOutput=off  UpperSaturationLimit=inf  LowerSaturationLimit=-inf  LinearizeAsGain=off  AntiWindupMode=none  Kb=1  TrackingMode=off  Kt=1  PParamMin=[]  PParamMax=[]  IParamMin=[]  IParamMax=[]  DParamMin=[]  DParamMax=[]  NParamMin=[]  NParamMax=[]  KbParamMin=[]  KbParamMax=[]  KtParamMin=[]  KtParamMax=[]  POutMin=[]  POutMax=[]  IOutMin=[]  IOutMax=[]  DOutMin=[]  DOutMax=[]  NOutMin=[]  NOutMax=[]  KbOutMin=[]  KbOutMax=[]  KtOutMin=[]  KtOutMax=[]  IntegratorOutMin=[]  IntegratorOutMax=[]  FilterOutMin=[]  FilterOutMax=[]  SumOutMin=[]  SumOutMax=[]  SumI1OutMin=[]  SumI1OutMax=[]  SumI2OutMin=[]  SumI2OutMax=[]  SumI3OutMin=[]  SumI3OutMax=[]  SumDOutMin=[]  SumDOutMax=[]  SaturationOutMin=[]  SaturationOutMax=[]  IntegratorContinuousStateAttributes=''  IntegratorStateMustResolveToSignalObject=off  IntegratorRTWStateStorageClass=Auto  FilterContinuousStateAttributes=''  FilterStateMustResolveToSignalObject=off  FilterRTWStateStorageClass=Auto  DifferentiatorICPrevScaledInput=0  DifferentiatorOutMin=[]  DifferentiatorOutMax=[]  InitialConditionSetting=State (most efficient)  FilterDiffOutCoefMin=[]  FilterDiffOutCoefMax=[]  SumDenOutMin=[]  SumDenOutMax=[]  SumNumOutMin=[]  SumNumOutMax=[]  ReciprocalOutMin=[]  ReciprocalOutMax=[]  DivideOutMin=[]  DivideOutMax=[]  TunerSelectOption=Transfer Function Based (PID Tuner App)
  Discrete PID Controller{1..5} (5 alike) : simulink/Continuous/PID Controller  Controller=PID  TimeDomain=Discrete-time  SampleTime=-1  IntegratorMethod=Forward Euler  FilterMethod=Forward Euler  Form=Parallel  UseFilter=on  ControllerParametersSource=internal  P=1  I=1  D=0  N=100  InitialConditionSource=internal  InitialConditionForIntegrator=0  InitialConditionForFilter=0  ExternalReset=none  LimitOutput=off  UpperSaturationLimit=inf  LowerSaturationLimit=-inf  LinearizeAsGain=off  AntiWindupMode=none  Kb=1  TrackingMode=off  Kt=1  PParamMin=[]  PParamMax=[]  IParamMin=[]  IParamMax=[]  DParamMin=[]  DParamMax=[]  NParamMin=[]  NParamMax=[]  KbParamMin=[]  KbParamMax=[]  KtParamMin=[]  KtParamMax=[]  POutMin=[]  POutMax=[]  IOutMin=[]  IOutMax=[]  DOutMin=[]  DOutMax=[]  NOutMin=[]  NOutMax=[]  KbOutMin=[]  KbOutMax=[]  KtOutMin=[]  KtOutMax=[]  IntegratorOutMin=[]  IntegratorOutMax=[]  FilterOutMin=[]  FilterOutMax=[]  SumOutMin=[]  SumOutMax=[]  SumI1OutMin=[]  SumI1OutMax=[]  SumI2OutMin=[]  SumI2OutMax=[]  SumI3OutMin=[]  SumI3OutMax=[]  SumDOutMin=[]  SumDOutMax=[]  SaturationOutMin=[]  SaturationOutMax=[]  IntegratorContinuousStateAttributes=''  IntegratorStateMustResolveToSignalObject=off  IntegratorRTWStateStorageClass=Auto  FilterContinuousStateAttributes=''  FilterStateMustResolveToSignalObject=off  FilterRTWStateStorageClass=Auto  DifferentiatorICPrevScaledInput=0  DifferentiatorOutMin=[]  DifferentiatorOutMax=[]  InitialConditionSetting=State (most efficient)  FilterDiffOutCoefMin=[]  FilterDiffOutCoefMax=[]  SumDenOutMin=[]  SumDenOutMax=[]  SumNumOutMin=[]  SumNumOutMax=[]  ReciprocalOutMin=[]  ReciprocalOutMax=[]  DivideOutMin=[]  DivideOutMax=[]  TunerSelectOption=Transfer Function Based (PID Tuner App)
  Subtract{,1..5} (6 alike) : Sum  Inputs=+-
  beta_ref : Constant  Value=beta_ref
  ref_velocity : Constant  Value=vx
  yawrate_ref : Constant  Value=vx/r
  cmd_offset : Outport
  cmd_yawAcc_beta : Outport  Port=2
  cmd_yawAcc_yawRate : Outport  Port=3
  cmd_velocity : Outport  Port=4
  wires:
  Discrete PID Controller5/1 -> cmd_velocity/1  "cmd_velocity"
  Subtract5/1 -> Discrete PID Controller5/1
  ref_velocity/1 -> Subtract5/1
  [vel_X] -> Subtract5/2
  Discrete Derivative/1 -> Subtract2/2, Subtract4/2
  Constant4/1 -> Subtract3/1  "ref_offset"
  Discrete PID Controller3/1 -> cmd_yawAcc_beta/1  "cmd_yawAcc_beta"
  Subtract/1 -> Discrete PID Controller1/1  "beta_error"
  Subtract4/1 -> Discrete PID Controller4/1
  beta_ref/1 -> Subtract/1
  Discrete PID Controller2/1 -> Subtract4/1  "yawAcc_ref2"
  Subtract3/1 -> Discrete PID Controller/1  "offset_error"
  [yawRate] -> Subtract1/2, Discrete Derivative/1
  Discrete PID Controller1/1 -> Subtract2/1  "yawAcc_ref1"
  yawrate_ref/1 -> Subtract1/1
  Subtract2/1 -> Discrete PID Controller3/1
  [offset_Lateral] -> Subtract3/2
  Discrete PID Controller/1 -> cmd_offset/1  "cmd_offset"
  [beta] -> Subtract/2
  Subtract1/1 -> Discrete PID Controller2/1  "yawRate_error"
  Discrete PID Controller4/1 -> cmd_yawAcc_yawRate/1  "cmd_yawAcc_yawRate"

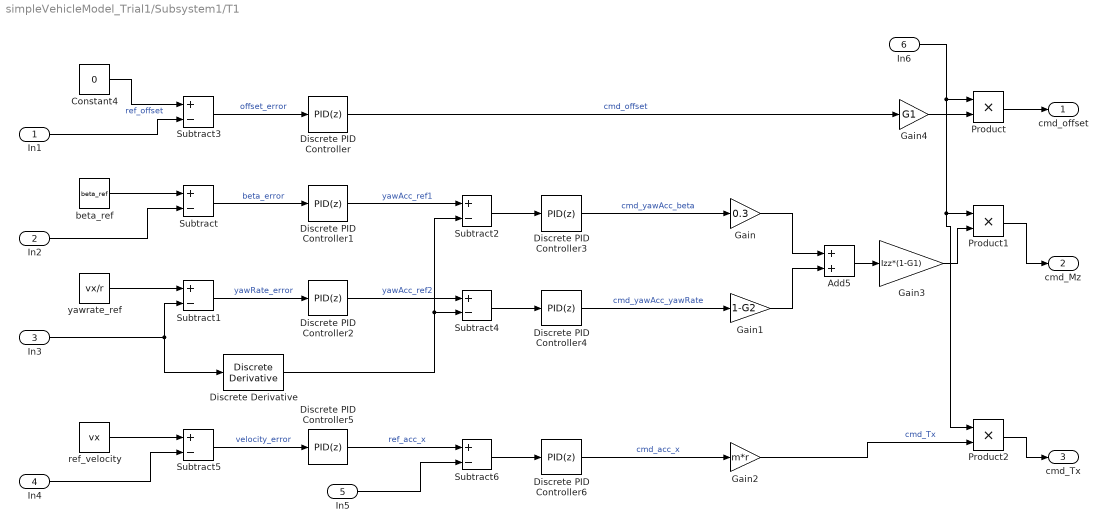
== system simpleVehicleModel_Trial1/Subsystem1/T1 ==
  In1 : Inport
  In2 : Inport  Port=2
  In3 : Inport  Port=3
  In4 : Inport  Port=4
  In5 : Inport  Port=5
  In6 : Inport  Port=6
  Add5 : Sum
  Constant4 : Constant  Value=0
  Discrete Derivative : simulink/Discrete/Discrete Derivative  gainval=1.0  ICPrevScaledInput=0.0  OutMin=[]  OutMax=[]  OutDataType=fixdt(1, 16)  OutScaling=2^-10  DoSatur=off
  Discrete PID Controller : simulink/Continuous/PID Controller  Controller=PID  TimeDomain=Discrete-time  SampleTime=-1  IntegratorMethod=Forward Euler  FilterMethod=Forward Euler  Form=Parallel  UseFilter=on  ControllerParametersSource=internal  P=1  I=0  D=0.1  N=100  InitialConditionSource=internal  InitialConditionForIntegrator=0  InitialConditionForFilter=0  ExternalReset=none  LimitOutput=off  UpperSaturationLimit=inf  LowerSaturationLimit=-inf  LinearizeAsGain=off  AntiWindupMode=none  Kb=1  TrackingMode=off  Kt=1  PParamMin=[]  PParamMax=[]  IParamMin=[]  IParamMax=[]  DParamMin=[]  DParamMax=[]  NParamMin=[]  NParamMax=[]  KbParamMin=[]  KbParamMax=[]  KtParamMin=[]  KtParamMax=[]  POutMin=[]  POutMax=[]  IOutMin=[]  IOutMax=[]  DOutMin=[]  DOutMax=[]  NOutMin=[]  NOutMax=[]  KbOutMin=[]  KbOutMax=[]  KtOutMin=[]  KtOutMax=[]  IntegratorOutMin=[]  IntegratorOutMax=[]  FilterOutMin=[]  FilterOutMax=[]  SumOutMin=[]  SumOutMax=[]  SumI1OutMin=[]  SumI1OutMax=[]  SumI2OutMin=[]  SumI2OutMax=[]  SumI3OutMin=[]  SumI3OutMax=[]  SumDOutMin=[]  SumDOutMax=[]  SaturationOutMin=[]  SaturationOutMax=[]  IntegratorContinuousStateAttributes=''  IntegratorStateMustResolveToSignalObject=off  IntegratorRTWStateStorageClass=Auto  FilterContinuousStateAttributes=''  FilterStateMustResolveToSignalObject=off  FilterRTWStateStorageClass=Auto  DifferentiatorICPrevScaledInput=0  DifferentiatorOutMin=[]  DifferentiatorOutMax=[]  InitialConditionSetting=State (most efficient)  FilterDiffOutCoefMin=[]  FilterDiffOutCoefMax=[]  SumDenOutMin=[]  SumDenOutMax=[]  SumNumOutMin=[]  SumNumOutMax=[]  ReciprocalOutMin=[]  ReciprocalOutMax=[]  DivideOutMin=[]  DivideOutMax=[]  TunerSelectOption=Transfer Function Based (PID Tuner App)
  Discrete PID Controller{1..6} (6 alike) : simulink/Continuous/PID Controller  Controller=PID  TimeDomain=Discrete-time  SampleTime=-1  IntegratorMethod=Forward Euler  FilterMethod=Forward Euler  Form=Parallel  UseFilter=on  ControllerParametersSource=internal  P=1  I=1  D=0  N=100  InitialConditionSource=internal  InitialConditionForIntegrator=0  InitialConditionForFilter=0  ExternalReset=none  LimitOutput=off  UpperSaturationLimit=inf  LowerSaturationLimit=-inf  LinearizeAsGain=off  AntiWindupMode=none  Kb=1  TrackingMode=off  Kt=1  PParamMin=[]  PParamMax=[]  IParamMin=[]  IParamMax=[]  DParamMin=[]  DParamMax=[]  NParamMin=[]  NParamMax=[]  KbParamMin=[]  KbParamMax=[]  KtParamMin=[]  KtParamMax=[]  POutMin=[]  POutMax=[]  IOutMin=[]  IOutMax=[]  DOutMin=[]  DOutMax=[]  NOutMin=[]  NOutMax=[]  KbOutMin=[]  KbOutMax=[]  KtOutMin=[]  KtOutMax=[]  IntegratorOutMin=[]  IntegratorOutMax=[]  FilterOutMin=[]  FilterOutMax=[]  SumOutMin=[]  SumOutMax=[]  SumI1OutMin=[]  SumI1OutMax=[]  SumI2OutMin=[]  SumI2OutMax=[]  SumI3OutMin=[]  SumI3OutMax=[]  SumDOutMin=[]  SumDOutMax=[]  SaturationOutMin=[]  SaturationOutMax=[]  IntegratorContinuousStateAttributes=''  IntegratorStateMustResolveToSignalObject=off  IntegratorRTWStateStorageClass=Auto  FilterContinuousStateAttributes=''  FilterStateMustResolveToSignalObject=off  FilterRTWStateStorageClass=Auto  DifferentiatorICPrevScaledInput=0  DifferentiatorOutMin=[]  DifferentiatorOutMax=[]  InitialConditionSetting=State (most efficient)  FilterDiffOutCoefMin=[]  FilterDiffOutCoefMax=[]  SumDenOutMin=[]  SumDenOutMax=[]  SumNumOutMin=[]  SumNumOutMax=[]  ReciprocalOutMin=[]  ReciprocalOutMax=[]  DivideOutMin=[]  DivideOutMax=[]  TunerSelectOption=Transfer Function Based (PID Tuner App)
  Gain : Gain  Gain=0.3
  Gain1 : Gain  Gain=1-G2
  Gain2 : Gain  Gain=m*r
  Gain3 : Gain  Gain=Izz*(1-G1)
  Gain4 : Gain  Gain=G1
  Product : Product
  Product1 : Product
  Product2 : Product
  Subtract{,1..6} (7 alike) : Sum  Inputs=+-
  beta_ref : Constant  Value=beta_ref
  ref_velocity : Constant  Value=vx
  yawrate_ref : Constant  Value=vx/r
  cmd_offset : Outport
  cmd_Mz : Outport  Port=2
  cmd_Tx : Outport  Port=3
  wires:
  Discrete PID Controller4/1 -> Gain1/1  "cmd_yawAcc_yawRate"
  Subtract1/1 -> Discrete PID Controller2/1  "yawRate_error"
  In2/1 -> Subtract/2
  Discrete PID Controller/1 -> Gain4/1  "cmd_offset"
  In1/1 -> Subtract3/2
  Subtract2/1 -> Discrete PID Controller3/1
  yawrate_ref/1 -> Subtract1/1
  Discrete PID Controller1/1 -> Subtract2/1  "yawAcc_ref1"
  In3/1 -> Discrete Derivative/1, Subtract1/2
  Subtract3/1 -> Discrete PID Controller/1  "offset_error"
  Discrete PID Controller2/1 -> Subtract4/1  "yawAcc_ref2"
  beta_ref/1 -> Subtract/1
  Subtract4/1 -> Discrete PID Controller4/1
  Subtract/1 -> Discrete PID Controller1/1  "beta_error"
  Discrete PID Controller3/1 -> Gain/1  "cmd_yawAcc_beta"
  Constant4/1 -> Subtract3/1  "ref_offset"
  Discrete Derivative/1 -> Subtract4/2, Subtract2/2
  In4/1 -> Subtract5/2
  ref_velocity/1 -> Subtract5/1
  Subtract5/1 -> Discrete PID Controller5/1  "velocity_error"
  Discrete PID Controller5/1 -> Subtract6/1  "ref_acc_x"
  Gain1/1 -> Add5/2
  Gain/1 -> Add5/1
  Add5/1 -> Gain3/1
  Subtract6/1 -> Discrete PID Controller6/1
  In5/1 -> Subtract6/2
  Discrete PID Controller6/1 -> Gain2/1  "cmd_acc_x"
  Product/1 -> cmd_offset/1
  In6/1 -> Product2/1, Product1/1, Product/1
  Gain4/1 -> Product/2
  Product1/1 -> cmd_Mz/1
  Product2/1 -> cmd_Tx/1
  Gain2/1 -> Product2/2  "cmd_Tx"
  Gain3/1 -> Product1/2

== system simpleVehicleModel_Trial1/Subsystem1/Track Segment Identifier ==
  1 if in first straight : Subsystem
  1 if in first turn : Subsystem
  1 if in last straight : Subsystem
  1 if in second turn : Subsystem
  1 if in transition phase : Subsystem
  Scope : Scope  NumInputPorts=5
  Out1 : Outport
  Out2 : Outport  Port=2
  Out3 : Outport  Port=3
  Out4 : Outport  Port=4
  Out5 : Outport  Port=5
  tag scope: S1=global, S2=global, S3=global, T1=global, T2=global
  wires:
  1 if in first turn/1(check turn 1) -> Scope/2, Out2/1, [T1]
  1 if in second turn/1(check turn 2) -> Scope/4, Out4/1, [T2]
  1 if in last straight/1(check last straight) -> Out5/1, [S3], Scope/5
  1 if in first straight/1(check straight 1) -> Scope/1, Out1/1, [S1]
  1 if in transition phase/1(check transition) -> Scope/3, Out3/1, [S2]

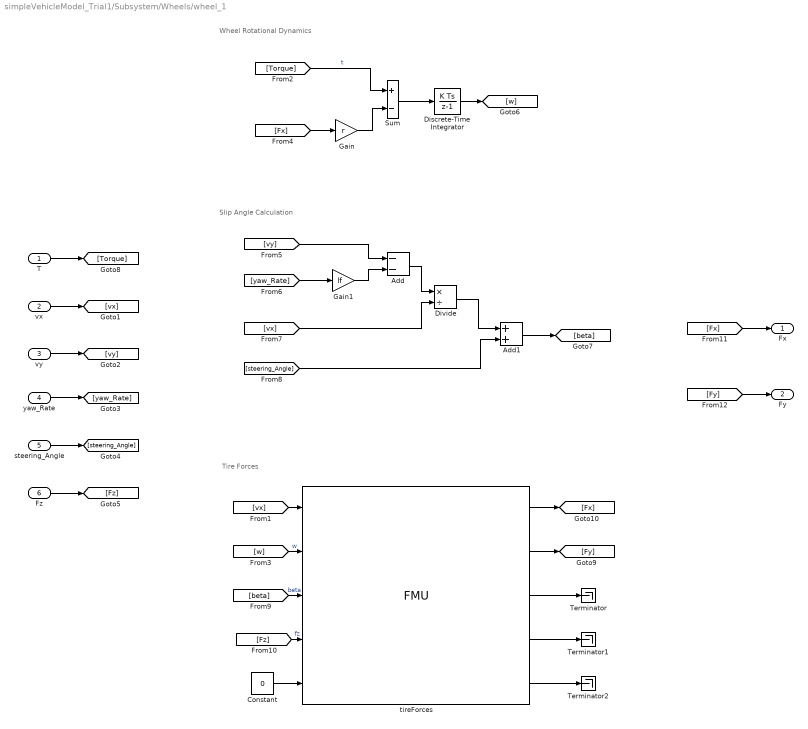
== system simpleVehicleModel_Trial1/Subsystem/Wheels/wheel_1 ==
  note: Tire Forces
  note: Wheel Rotational Dynamics
  note: Slip Angle Calculation
  T : Inport
  vx : Inport  Port=2
  vy : Inport  Port=3
  yaw_Rate : Inport  Port=4
  steering_Angle : Inport  Port=5
  Fz : Inport  Port=6
  Add : Sum  Inputs=--
  Add1 : Sum
  Constant : Constant  Value=0
  Discrete-Time Integrator : DiscreteIntegrator  InitialConditionSetting=State (most efficient)  SampleTime=-1  ICPrevOutput=DiscIntNeverNeededParam  ICPrevScaledInput=DiscIntNeverNeededParam
  Divide : Product  Inputs=*/
  Gain : Gain  Gain=r
  Gain1 : Gain  Gain=lf
  Sum : Sum  Inputs=+-
  Terminator : Terminator
  Terminator1 : Terminator
  Terminator2 : Terminator
  tireForces : FMU  FMUName=MED2018_TireModel.fmu  FMUMode=CoSimulation  FMUSampleTime=-1  mask(TyreFMUContainer [Co-Simulation, v2.0]){}
      mask Display:
      | disp('TyreFMUContainer');
      | port_label('output',1,'Fx');
      | port_label('output',2,'Fy');
      | port_label('output',3,'Mz');
      | port_label('output',4,'r');
      | port_label('output',5,'Mx');
      | port_label('input',1,'vx');
      | port_label('input',2,'w');
      | port_label('input',3,'beta');
      | port_label('input',4,'Fz');
      | port_label('input',5,'camber');
  Fx : Outport
  Fy : Outport  Port=2
  wires:
  Discrete-Time Integrator/1 -> [w]
  tireForces/5 -> Terminator2/1
  tireForces/2 -> [Fy]
  tireForces/4 -> Terminator1/1
  tireForces/3 -> Terminator/1
  Sum/1 -> Discrete-Time Integrator/1
  [Torque] -> Sum/1  "t"
  Gain/1 -> Sum/2
  [Fx] -> Gain/1
  Constant/1 -> tireForces/5
  Gain1/1 -> Add/2
  Add/1 -> Divide/1
  [w] -> tireForces/2  "w"
  vx/1 -> [vx]
  vy/1 -> [vy]
  steering_Angle/1 -> [steering_Angle]
  yaw_Rate/1 -> [yaw_Rate]
  Fz/1 -> [Fz]
  [vx] -> tireForces/1
  [vy] -> Add/1
  [yaw_Rate] -> Gain1/1
  [vx] -> Divide/2
  Divide/1 -> Add1/1
  [steering_Angle] -> Add1/2
  Add1/1 -> [beta]
  [beta] -> tireForces/3  "beta"
  [Fz] -> tireForces/4  "fz"
  T/1 -> [Torque]
  tireForces/1 -> [Fx]
  [Fx] -> Fx/1
  [Fy] -> Fy/1

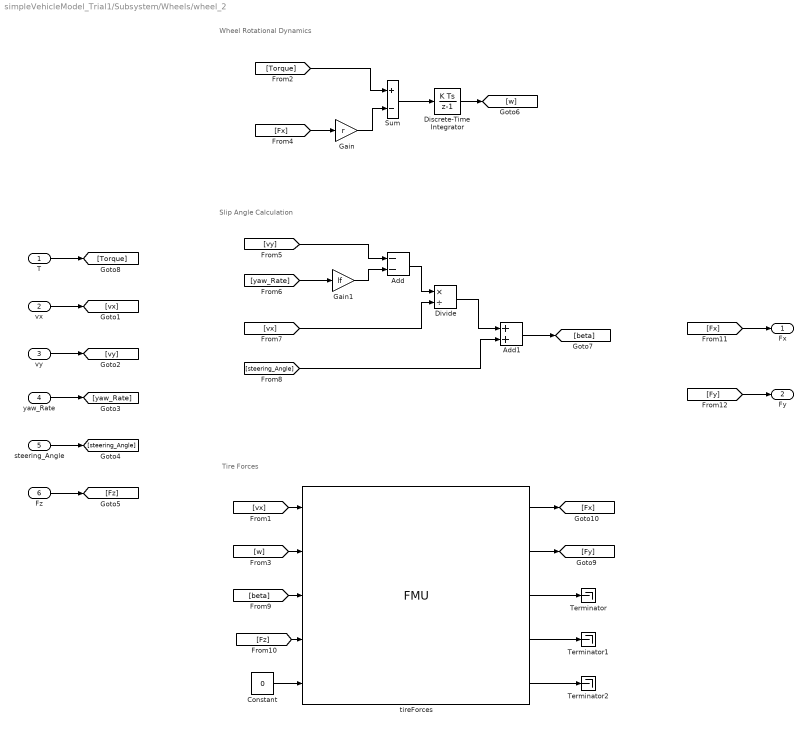
== system simpleVehicleModel_Trial1/Subsystem/Wheels/wheel_2 ==
  note: Tire Forces
  note: Wheel Rotational Dynamics
  note: Slip Angle Calculation
  T : Inport
  vx : Inport  Port=2
  vy : Inport  Port=3
  yaw_Rate : Inport  Port=4
  steering_Angle : Inport  Port=5
  Fz : Inport  Port=6
  Add : Sum  Inputs=--
  Add1 : Sum
  Constant : Constant  Value=0
  Discrete-Time Integrator : DiscreteIntegrator  InitialConditionSetting=State (most efficient)  SampleTime=-1  ICPrevOutput=DiscIntNeverNeededParam  ICPrevScaledInput=DiscIntNeverNeededParam
  Divide : Product  Inputs=*/
  Gain : Gain  Gain=r
  Gain1 : Gain  Gain=lf
  Sum : Sum  Inputs=+-
  Terminator : Terminator
  Terminator1 : Terminator
  Terminator2 : Terminator
  tireForces : FMU  FMUName=MED2018_TireModel.fmu  FMUMode=CoSimulation  FMUSampleTime=-1  mask(TyreFMUContainer [Co-Simulation, v2.0]){}
      mask Display:
      | disp('TyreFMUContainer');
      | port_label('output',1,'Fx');
      | port_label('output',2,'Fy');
      | port_label('output',3,'Mz');
      | port_label('output',4,'r');
      | port_label('output',5,'Mx');
      | port_label('input',1,'vx');
      | port_label('input',2,'w');
      | port_label('input',3,'beta');
      | port_label('input',4,'Fz');
      | port_label('input',5,'camber');
  Fx : Outport
  Fy : Outport  Port=2
  wires:
  Discrete-Time Integrator/1 -> [w]
  tireForces/5 -> Terminator2/1
  tireForces/2 -> [Fy]
  tireForces/4 -> Terminator1/1
  tireForces/3 -> Terminator/1
  Sum/1 -> Discrete-Time Integrator/1
  [Torque] -> Sum/1
  Gain/1 -> Sum/2
  [Fx] -> Gain/1
  Constant/1 -> tireForces/5
  Gain1/1 -> Add/2
  Add/1 -> Divide/1
  [w] -> tireForces/2
  vx/1 -> [vx]
  vy/1 -> [vy]
  steering_Angle/1 -> [steering_Angle]
  yaw_Rate/1 -> [yaw_Rate]
  Fz/1 -> [Fz]
  [vx] -> tireForces/1
  [vy] -> Add/1
  [yaw_Rate] -> Gain1/1
  [vx] -> Divide/2
  Divide/1 -> Add1/1
  [steering_Angle] -> Add1/2
  Add1/1 -> [beta]
  [beta] -> tireForces/3
  [Fz] -> tireForces/4
  T/1 -> [Torque]
  tireForces/1 -> [Fx]
  [Fx] -> Fx/1
  [Fy] -> Fy/1

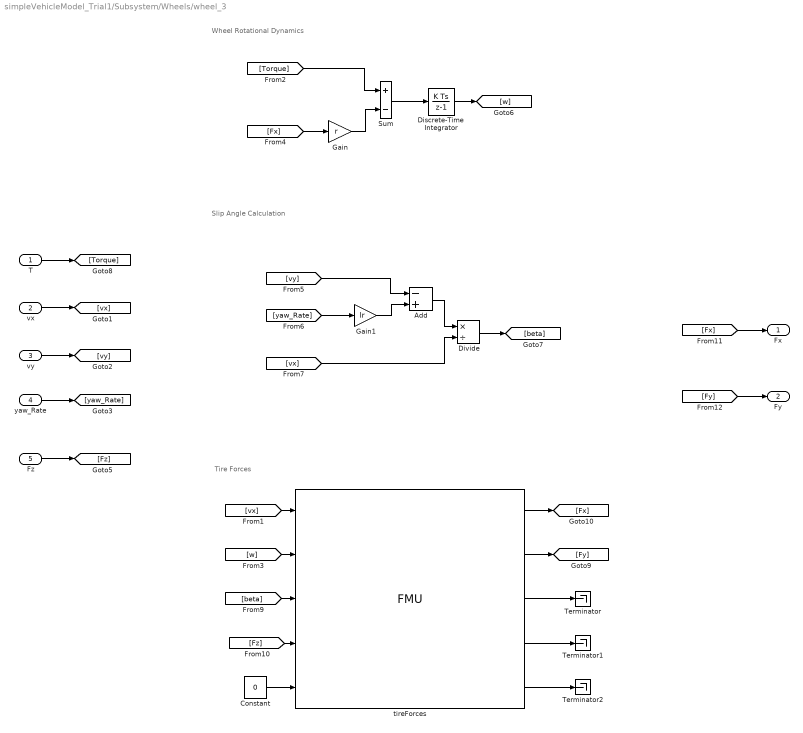
== system simpleVehicleModel_Trial1/Subsystem/Wheels/wheel_3 ==
  note: Tire Forces
  note: Wheel Rotational Dynamics
  note: Slip Angle Calculation
  T : Inport
  vx : Inport  Port=2
  vy : Inport  Port=3
  yaw_Rate : Inport  Port=4
  Fz : Inport  Port=5
  Add : Sum  Inputs=-+
  Constant : Constant  Value=0
  Discrete-Time Integrator : DiscreteIntegrator  InitialConditionSetting=State (most efficient)  SampleTime=-1  ICPrevOutput=DiscIntNeverNeededParam  ICPrevScaledInput=DiscIntNeverNeededParam
  Divide : Product  Inputs=*/
  Gain : Gain  Gain=r
  Gain1 : Gain  Gain=lr
  Sum : Sum  Inputs=+-
  Terminator : Terminator
  Terminator1 : Terminator
  Terminator2 : Terminator
  tireForces : FMU  FMUName=MED2018_TireModel.fmu  FMUMode=CoSimulation  FMUSampleTime=-1  mask(TyreFMUContainer [Co-Simulation, v2.0]){}
      mask Display:
      | disp('TyreFMUContainer');
      | port_label('output',1,'Fx');
      | port_label('output',2,'Fy');
      | port_label('output',3,'Mz');
      | port_label('output',4,'r');
      | port_label('output',5,'Mx');
      | port_label('input',1,'vx');
      | port_label('input',2,'w');
      | port_label('input',3,'beta');
      | port_label('input',4,'Fz');
      | port_label('input',5,'camber');
  Fx : Outport
  Fy : Outport  Port=2
  wires:
  Discrete-Time Integrator/1 -> [w]
  tireForces/5 -> Terminator2/1
  tireForces/2 -> [Fy]
  tireForces/4 -> Terminator1/1
  tireForces/3 -> Terminator/1
  Sum/1 -> Discrete-Time Integrator/1
  [Torque] -> Sum/1
  Gain/1 -> Sum/2
  [Fx] -> Gain/1
  Constant/1 -> tireForces/5
  Gain1/1 -> Add/2
  Add/1 -> Divide/1
  [w] -> tireForces/2
  vx/1 -> [vx]
  vy/1 -> [vy]
  yaw_Rate/1 -> [yaw_Rate]
  Fz/1 -> [Fz]
  [vx] -> tireForces/1
  [vy] -> Add/1
  [yaw_Rate] -> Gain1/1
  [vx] -> Divide/2
  [beta] -> tireForces/3
  [Fz] -> tireForces/4
  T/1 -> [Torque]
  tireForces/1 -> [Fx]
  [Fx] -> Fx/1
  [Fy] -> Fy/1
  Divide/1 -> [beta]

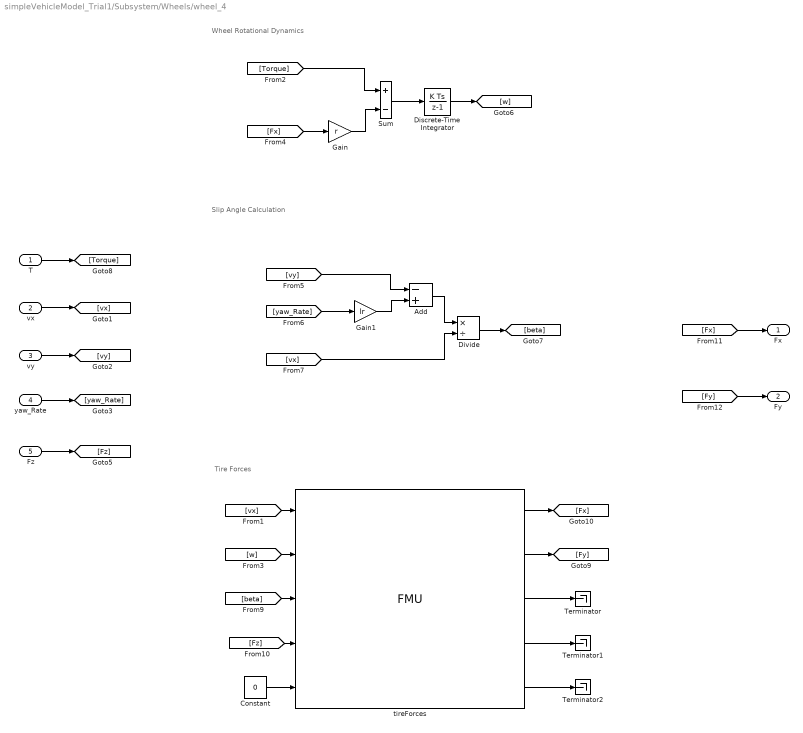
== system simpleVehicleModel_Trial1/Subsystem/Wheels/wheel_4 ==
  note: Tire Forces
  note: Wheel Rotational Dynamics
  note: Slip Angle Calculation
  T : Inport
  vx : Inport  Port=2
  vy : Inport  Port=3
  yaw_Rate : Inport  Port=4
  Fz : Inport  Port=5
  Add : Sum  Inputs=-+
  Constant : Constant  Value=0
  Discrete-Time Integrator : DiscreteIntegrator  InitialConditionSetting=State (most efficient)  SampleTime=-1  ICPrevOutput=DiscIntNeverNeededParam  ICPrevScaledInput=DiscIntNeverNeededParam
  Divide : Product  Inputs=*/
  Gain : Gain  Gain=r
  Gain1 : Gain  Gain=lr
  Sum : Sum  Inputs=+-
  Terminator : Terminator
  Terminator1 : Terminator
  Terminator2 : Terminator
  tireForces : FMU  FMUName=MED2018_TireModel.fmu  FMUDebugLogging=on  FMUMode=CoSimulation  FMUSampleTime=-1  mask(TyreFMUContainer [Co-Simulation, v2.0]){}
      mask Display:
      | disp('TyreFMUContainer');
      | port_label('output',1,'Fx');
      | port_label('output',2,'Fy');
      | port_label('output',3,'Mz');
      | port_label('output',4,'r');
      | port_label('output',5,'Mx');
      | port_label('input',1,'vx');
      | port_label('input',2,'w');
      | port_label('input',3,'beta');
      | port_label('input',4,'Fz');
      | port_label('input',5,'camber');
  Fx : Outport
  Fy : Outport  Port=2
  wires:
  Discrete-Time Integrator/1 -> [w]
  tireForces/5 -> Terminator2/1
  tireForces/2 -> [Fy]
  tireForces/4 -> Terminator1/1
  tireForces/3 -> Terminator/1
  Sum/1 -> Discrete-Time Integrator/1
  [Torque] -> Sum/1
  Gain/1 -> Sum/2
  [Fx] -> Gain/1
  Constant/1 -> tireForces/5
  [w] -> tireForces/2
  vx/1 -> [vx]
  vy/1 -> [vy]
  yaw_Rate/1 -> [yaw_Rate]
  Fz/1 -> [Fz]
  [vx] -> tireForces/1
  [beta] -> tireForces/3
  [Fz] -> tireForces/4
  T/1 -> [Torque]
  tireForces/1 -> [Fx]
  [Fx] -> Fx/1
  [Fy] -> Fy/1
  [vy] -> Add/1
  [vx] -> Divide/2
  [yaw_Rate] -> Gain1/1
  Add/1 -> Divide/1
  Gain1/1 -> Add/2
  Divide/1 -> [beta]
